simulink library "controlSim_Lib"  (R2021b)
settings: Solver=ode45  StartTime=0.0  StopTime=10.0  RelTol=1e-3  EnableMultiTasking=on
undefined symbols (not defined in the file or in its folder): controlSim, simu
settings Model: RequirementInfo="{}  %GIDa_42666abb_d6d9_408c_ae24_f6520282b61c"  Creator=sor  LastModifiedBy=jtgrasb
settings SolverCC: AlgebraicLoopSolver=TrustRegion
settings DataIOCC: LimitDataPoints=on  SaveFormat=Array  ReturnWorkspaceOutputs=off
settings OptimizationCC: LifeSpan=inf
settings DebuggingCC: SolverPrmCheckMsg=warning  AllowSymbolicDim=off  SFUnexpectedBacktrackingDiag=warning  SFNoUnconditionalDefaultTransitionDiag=warning  SFExecutionAtInitializationDiag=none  SFMachineParentedDataDiag=warning  ArithmeticOperatorsInVariantConditions=warning
settings HardwareCC: ProdBitPerPointer=32  ProdBitPerSizeT=32  ProdBitPerPtrDiffT=32  ProdLargestAtomicFloat=None  ProdIntDivRoundTo=Undefined  ProdEndianess=Unspecified  ProdWordSize=32  ProdHWDeviceType=32-bit Generic
settings ModelReferenceCC: PropagateSignalLabelsOutOfModel=off
settings SFSimCC: SimUseLocalCustomCode=off  CustomCodeUndefinedFunction=UseInterfaceOnly
settings RTWCC: RTWUseLocalCustomCode=off
settings CodeAppCC: StateflowObjectComments=on
settings GRTTargetCC: TargetLangStandard=C89/C90 (ANSI)
settings ConfigComp: CovMetricSettings=dw  CovSaveCumulativeToWorkspaceVar=on  CovSaveSingleToWorkspaceVar=on  CovExternalEMLEnable=off  CovSFcnEnable=off

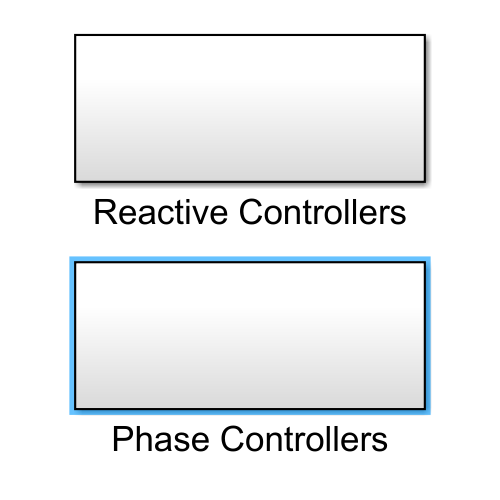
[thumbnail: Simulink's stored preview of the top-level diagram]
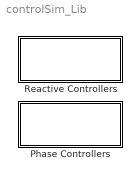
== system controlSim_Lib ==
  Phase Controllers : Subsystem
  Reactive Controllers : Subsystem

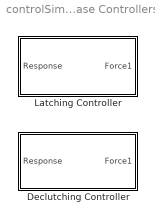
== system controlSim_Lib/Phase Controllers ==
  Declutching Controller : Subsystem  mask{controlSim=controlSim(1), InputFiletext=Use WEC-Sim input file to define Latching Controller parameters, Kp=0, Ki=0, declutchTime=0}
      mask prompts: controlSim "Declutching Controller"; Kp "Proportional gain (damping) [Ns/m]"; Ki "Integral gain (stiffness) [N/m]"; declutchTime "Declutching Time [s]"
      mask init:
      | if exist('controlSim','var')
      |     h=[gcb '/To Workspace'];
      |     responseName=['controlSim' num2str(controlSim.number) '_out'];
      |     set_param(h,'VariableName',responseName);
      | end
      | clear h responseName
      mask DialogControl CustomParameterGroup Prompt: Custom Parameters
      mask DialogControl DCParameters Prompt: Declutching Controller Parameters
  Latching Controller : Subsystem  mask{controlSim=controlSim(1), InputFiletext=Use WEC-Sim input file to define Latching Controller parameters, Kp=0, Ki=0, latchTime=0}
      mask prompts: controlSim "Latching Controller"; Kp "Proportional gain (damping) [Ns/m]"; Ki "Integral gain (stiffness) [N/m]"; latchTime "Latching Time [s]"
      mask init:
      | if exist('controlSim','var')
      |     h=[gcb '/To Workspace'];
      |     responseName=['controlSim' num2str(controlSim.number) '_out'];
      |     set_param(h,'VariableName',responseName);
      | end
      | clear h responseName
      mask DialogControl CustomParameterGroup Prompt: Custom Parameters
      mask DialogControl LCParameters Prompt: Latching Controller Parameters

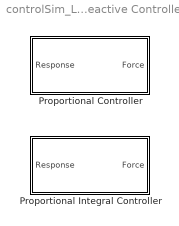
== system controlSim_Lib/Reactive Controllers ==
  Proportional Controller : Subsystem  mask{controlSim=controlSim(1), InputFiletext=Use WEC-Sim input file to define Latching Controller parameters, Kp=0}
      mask prompts: controlSim "Proportional Controller"; Kp "Proportional gain (damping) [Ns/m]"
      mask init:
      | if exist('controlSim','var')
      |     h=[gcb '/To Workspace'];
      |     responseName=['controlSim' num2str(controlSim.number) '_out'];
      |     set_param(h,'VariableName',responseName);
      | end
      | clear h responseName
      mask DialogControl CustomParameterGroup Prompt: Custom Parameters
      mask DialogControl PCParameters Prompt: Proportional Controller Parameters
  Proportional Integral Controller : Subsystem  mask{controlSim=controlSim(1), InputFiletext=Use WEC-Sim input file to define Latching Controller parameters, Kp=0, Ki=0}
      mask prompts: controlSim "Proportional Integral Controller"; Kp "Proportional gain (damping) [Ns/m]"; Ki "Integral gain (stiffness) [N/m]"
      mask init:
      | if exist('controlSim','var')
      |     h=[gcb '/To Workspace'];
      |     responseName=['controlSim' num2str(controlSim.number) '_out'];
      |     set_param(h,'VariableName',responseName);
      | end
      | clear h responseName
      mask DialogControl CustomParameterGroup Prompt: Custom Parameters
      mask DialogControl PICParameters Prompt: Proportional Integral Controller Parameters

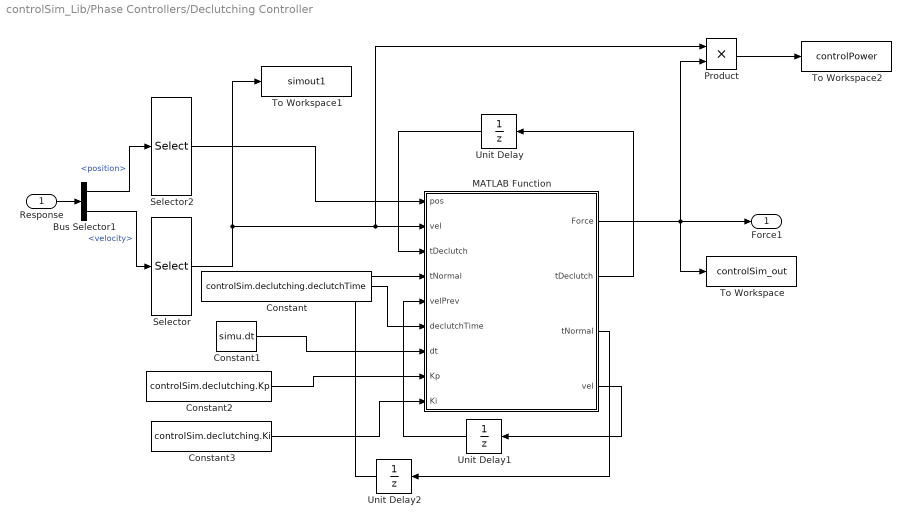
== system controlSim_Lib/Phase Controllers/Declutching Controller ==
  Response : Inport
  Bus Selector1 : BusSelector  OutputSignals=position,velocity
  Constant : Constant  Value=controlSim.declutching.declutchTime
  Constant1 : Constant  Value=simu.dt
  Constant2 : Constant  Value=controlSim.declutching.Kp
  Constant3 : Constant  Value=controlSim.declutching.Ki
  MATLAB Function : MATLAB Function  TreatAsAtomicUnit=on
  Product : Product
  Selector : Selector  InputPortWidth=6  IndexOptions=Index vector (dialog)  Indices=3  OutputSizes=1
  Selector2 : Selector  InputPortWidth=6  IndexOptions=Index vector (dialog)  Indices=3  OutputSizes=1
  To Workspace : ToWorkspace  VariableName=controlSim_out  SaveFormat=Timeseries  SampleTime=-1
  To Workspace1 : ToWorkspace  VariableName=simout1  SaveFormat=Timeseries  SampleTime=-1
  To Workspace2 : ToWorkspace  VariableName=controlPower  SaveFormat=Timeseries  SampleTime=-1
  Unit Delay : UnitDelay  SampleTime=-1  HasFrameUpgradeWarning=on
  Unit Delay1 : UnitDelay  SampleTime=-1  HasFrameUpgradeWarning=on
  Unit Delay2 : UnitDelay  SampleTime=-1  HasFrameUpgradeWarning=on
  Force1 : Outport
  wires:
  Selector2/1 -> MATLAB Function/1(pos)
  Product/1 -> To Workspace2/1
  Bus Selector1/1 -> Selector2/1  "<position>"
  Selector/1 -> To Workspace1/1, Product/1, MATLAB Function/2("vel ")
  Bus Selector1/2 -> Selector/1  "<velocity>"
  MATLAB Function/4(vel) -> Unit Delay1/1
  Unit Delay2/1 -> MATLAB Function/4("tNormal ")
  MATLAB Function/1(Force) -> Product/2, Force1/1, To Workspace/1
  Constant2/1 -> MATLAB Function/8(Kp)
  Unit Delay1/1 -> MATLAB Function/5(velPrev)
  Constant3/1 -> MATLAB Function/9(Ki)
  MATLAB Function/3(tNormal) -> Unit Delay2/1
  Constant/1 -> MATLAB Function/6(declutchTime)
  Unit Delay/1 -> MATLAB Function/3("tDeclutch ")
  Constant1/1 -> MATLAB Function/7(dt)
  MATLAB Function/2(tDeclutch) -> Unit Delay/1
  Response/1 -> Bus Selector1/1

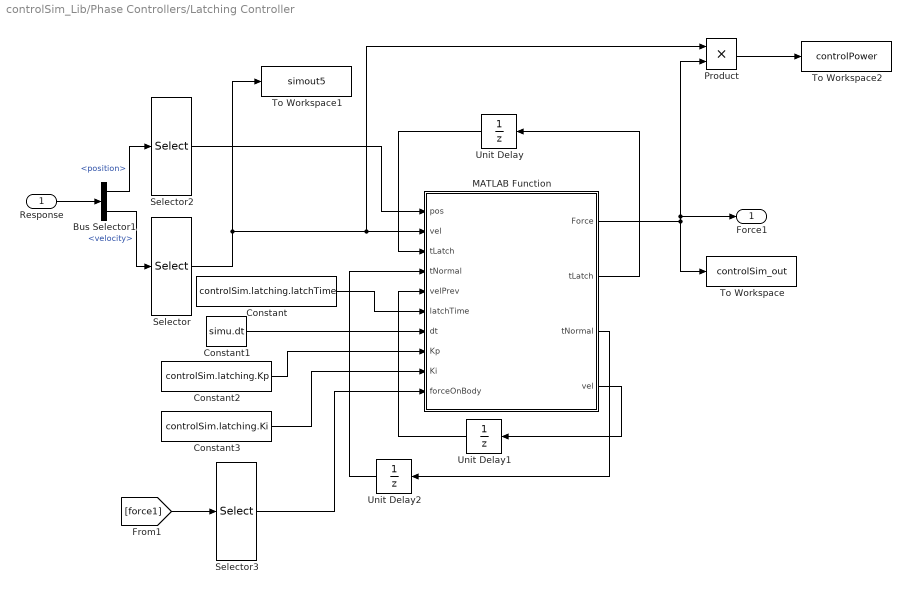
== system controlSim_Lib/Phase Controllers/Latching Controller ==
  Response : Inport
  Bus Selector1 : BusSelector  OutputSignals=position,velocity
  Constant : Constant  Value=controlSim.latching.latchTime
  Constant1 : Constant  Value=simu.dt
  Constant2 : Constant  Value=controlSim.latching.Kp
  Constant3 : Constant  Value=controlSim.latching.Ki
  MATLAB Function : MATLAB Function  TreatAsAtomicUnit=on
  Product : Product
  Selector : Selector  InputPortWidth=6  IndexOptions=Index vector (dialog)  Indices=3  OutputSizes=1
  Selector2 : Selector  InputPortWidth=6  IndexOptions=Index vector (dialog)  Indices=3  OutputSizes=1
  Selector3 : Selector  InputPortWidth=6  IndexOptions=Index vector (dialog)  Indices=3  OutputSizes=1
  To Workspace : ToWorkspace  VariableName=controlSim_out  SaveFormat=Timeseries  SampleTime=-1
  To Workspace1 : ToWorkspace  VariableName=simout5  SaveFormat=Timeseries  SampleTime=-1
  To Workspace2 : ToWorkspace  VariableName=controlPower  SaveFormat=Timeseries  SampleTime=-1
  Unit Delay : UnitDelay  SampleTime=-1  HasFrameUpgradeWarning=on
  Unit Delay1 : UnitDelay  SampleTime=-1  HasFrameUpgradeWarning=on
  Unit Delay2 : UnitDelay  SampleTime=-1  HasFrameUpgradeWarning=on
  Force1 : Outport
  wires:
  Constant1/1 -> MATLAB Function/7(dt)
  Response/1 -> Bus Selector1/1
  MATLAB Function/3(tNormal) -> Unit Delay2/1
  MATLAB Function/2(tLatch) -> Unit Delay/1
  Unit Delay2/1 -> MATLAB Function/4("tNormal ")
  Unit Delay1/1 -> MATLAB Function/5(velPrev)
  Unit Delay/1 -> MATLAB Function/3("tLatch ")
  Bus Selector1/2 -> Selector/1  "<velocity>"
  Constant/1 -> MATLAB Function/6(latchTime)
  Selector/1 -> To Workspace1/1, Product/1, MATLAB Function/2("vel ")
  MATLAB Function/4(vel) -> Unit Delay1/1
  MATLAB Function/1(Force) -> Product/2, Force1/1, To Workspace/1
  Bus Selector1/1 -> Selector2/1  "<position>"
  Selector2/1 -> MATLAB Function/1(pos)
  Selector3/1 -> MATLAB Function/10(forceOnBody)
  [force1] -> Selector3/1
  Constant3/1 -> MATLAB Function/9(Ki)
  Constant2/1 -> MATLAB Function/8(Kp)
  Product/1 -> To Workspace2/1

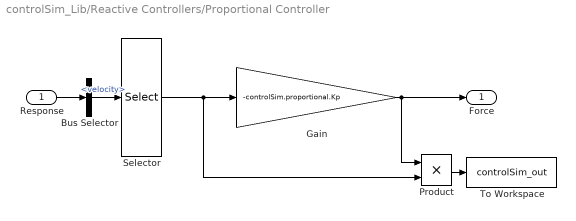
== system controlSim_Lib/Reactive Controllers/Proportional Controller ==
  Response : Inport
  Bus Selector : BusSelector  OutputSignals=velocity
  Gain : Gain  Gain=-controlSim.proportional.Kp
  Product : Product
  Selector : Selector  InputPortWidth=6  IndexOptions=Index vector (dialog)  Indices=[3]  OutputSizes=1
  To Workspace : ToWorkspace  VariableName=controlSim_out  SaveFormat=Timeseries  SampleTime=-1
  Force : Outport
  wires:
  Selector/1 -> Product/2, Gain/1
  Gain/1 -> Product/1, Force/1
  Product/1 -> To Workspace/1
  Response/1 -> Bus Selector/1
  Bus Selector/1 -> Selector/1  "<velocity>"

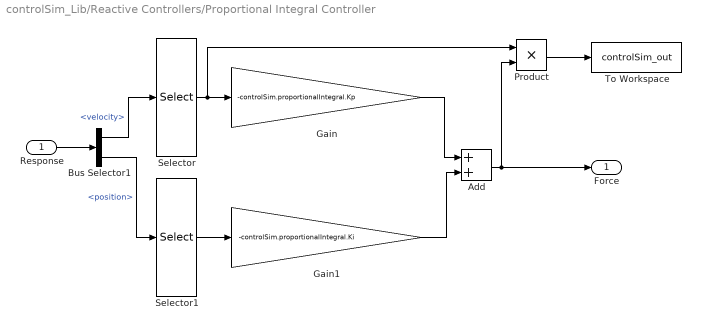
== system controlSim_Lib/Reactive Controllers/Proportional Integral Controller ==
  Response : Inport
  Add : Sum
  Bus Selector1 : BusSelector  OutputSignals=velocity,position
  Gain : Gain  Gain=-controlSim.proportionalIntegral.Kp
  Gain1 : Gain  Gain=-controlSim.proportionalIntegral.Ki
  Product : Product
  Selector : Selector  InputPortWidth=6  IndexOptions=Index vector (dialog)  Indices=[3]  OutputSizes=1
  Selector1 : Selector  InputPortWidth=6  IndexOptions=Index vector (dialog)  Indices=[3]  OutputSizes=1
  To Workspace : ToWorkspace  VariableName=controlSim_out  SaveFormat=Timeseries  SampleTime=-1
  Force : Outport
  wires:
  Selector/1 -> Gain/1, Product/1
  Selector1/1 -> Gain1/1
  Gain1/1 -> Add/2
  Add/1 -> Product/2, Force/1
  Gain/1 -> Add/1
  Product/1 -> To Workspace/1
  Response/1 -> Bus Selector1/1
  Bus Selector1/1 -> Selector/1  "<velocity>"
  Bus Selector1/2 -> Selector1/1  "<position>"

== matlab function controlSim_Lib/Phase Controllers/Latching Controller/MATLAB Function ==
  data: pos input; vel input; Force output; tLatch input; tNormal input; velPrev input; tLatch output; tNormal output; vel output; latchTime input; dt input; Kp input; Ki input; forceOnBody input
function [Force, tLatch, tNormal, vel] = fcn(pos, vel, tLatch, tNormal, velPrev, latchTime, dt, Kp, Ki, forceOnBody)

if ((diff(sign([vel,velPrev]))~=0 && tLatch==0 && tNormal>.2) || (tLatch>0 && tLatch<latchTime))
    Force = -forceOnBody;
    tLatch = tLatch + dt;
    tNormal = 0;
else
    Force = -Kp*vel + -Ki*pos;
    tNormal = tNormal + dt;
    tLatch = 0;
end
end

== matlab function controlSim_Lib/Phase Controllers/Declutching Controller/MATLAB Function ==
  data: pos input; vel input; Force output; tDeclutch input; tNormal input; velPrev input; tDeclutch output; tNormal output; vel output; declutchTime input; dt input; Kp input; Ki input
function [Force, tDeclutch, tNormal, vel] = fcn(pos, vel, tDeclutch, tNormal, velPrev, declutchTime, dt, Kp, Ki)

if ((diff(sign([vel,velPrev]))~=0 && tDeclutch==0 && tNormal>.2) || (tDeclutch>0 && tDeclutch<declutchTime))
    Force = 0;
    tDeclutch = tDeclutch + dt;
    tNormal = 0;
else
    Force = -Kp*vel + -Ki*pos;
    tNormal = tNormal + dt;
    tDeclutch = 0;
end
end
